simulink model "Sim3DoF"  (R2025b)
settings: Solver=VariableStepAuto  StartTime=0.0  StopTime=36  RelTol=1e-3
values from neighbouring files (symbols this model uses):
  hiddenLayerSizeCtrl = (2 * inputLayerSizeCtrl + 1) * 1    (= 13)    [Init2DoF.m]    (also in Init3DoF.m = 3)
  hiddenLayerSizeObsv = (2 * inputLayerSizeObsv + 1) * 1    (= 17)    [Init2DoF.m]    (also in Init3DoF.m = 3)
  n = 4    [Init2DoF.m]    (also in Init3DoF.m = 6)
  u_max = 12 * [1; 0.8]    [Init2DoF.m]    (also in Init3DoF.m = 25 * [1; 1; 1])
  u_min = - 12 * [1; 0.8]    [Init2DoF.m]    (also in Init3DoF.m = - 25 * [1; 1; 1])
  Vctrl0 = 0.1 * randn(hiddenLayerSizeCtrl, inputLayerSizeCtrl)    [Init2DoF.m]    (also in Init3DoF.m)
  Vobsv0 = 0.1 * randn(hiddenLayerSizeObsv, inputLayerSizeObsv)    [Init2DoF.m]    (also in Init3DoF.m)
  Wctrl0 = 0.1 * randn(outputLayerSizeCtrl, hiddenLayerSizeCtrl)    [Init2DoF.m]    (also in Init3DoF.m)
  Wobsv0 = 0.1 * randn(outputLayerSizeObsv, hiddenLayerSizeObsv)    [Init2DoF.m]    (also in Init3DoF.m)
  x0 = [0; 0.5; 0.1; 0]    [Init2DoF.m]    (also in Init3DoF.m = zeros(n, 1))
  x_hat0 = x0([1, 3, 2, 4])    [Init2DoF.m]    (also in Init3DoF.m = zeros(n, 1))
libraries: eeGeneralControl x2
settings Model: Creator=Asus  LastModifiedBy=Asus

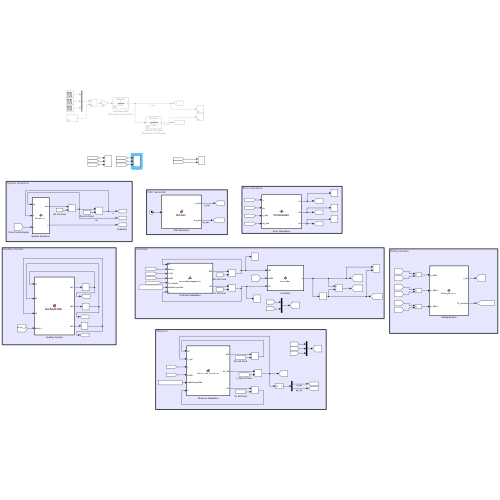
[thumbnail: Simulink's stored preview of the top-level diagram]
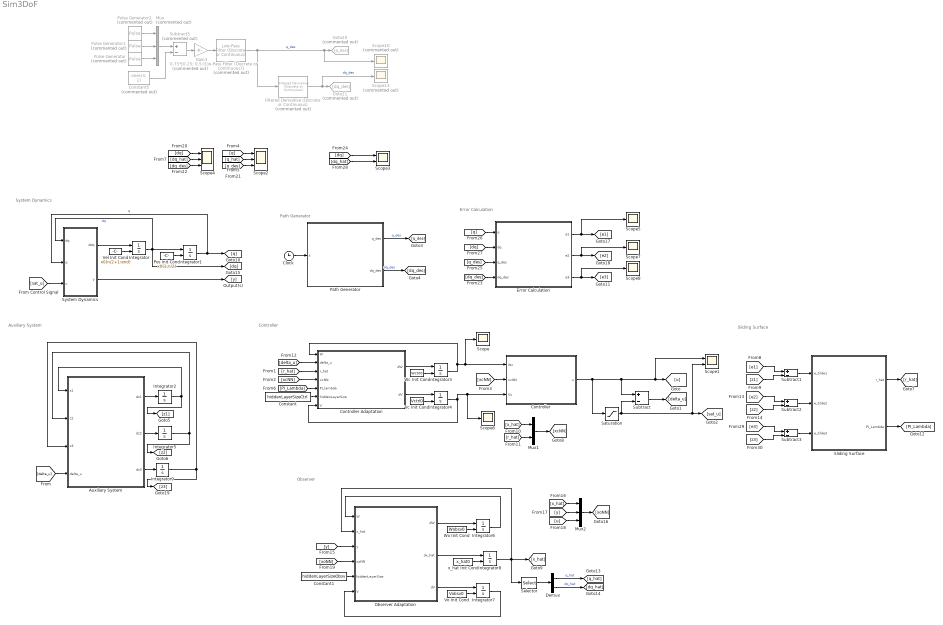
== system Sim3DoF ==
  note: System Dynamics
  note: Path Generator
  note: Auxiliary System
  note: Controller
  note: Sliding Surface
  note: Observer
  note: Error Calculation
  Auxiliary System : MATLAB Function  TreatAsAtomicUnit=on
  Clock : Clock
  Constant : Constant  Value=hiddenLayerSizeCtrl
  Constant1 : Constant  Value=hiddenLayerSizeObsv
  Constant5 : Constant  Commented=on  Value=ones(3, 1)
  Controller : MATLAB Function  TreatAsAtomicUnit=on
  Controller Adaptation : MATLAB Function  TreatAsAtomicUnit=on
  Demux : Demux  Outputs=2
  Error Calculation : MATLAB Function  TreatAsAtomicUnit=on
  Filtered Derivative (Discrete or Continuous) : eeGeneralControl/Filtered Derivative (Discrete or Continuous)  Commented=on  K=1  T=0.01  B=inf  A=-inf  minRatio=10  init_option=Inherited from block input  x0=0  Ts=-1
      settings: LibrarySourceBlock=|
      | ee_sl_lib/General Control/Filtered Derivative
      | (Discrete or Continuous)
  Gain3 : Gain  Commented=on  Gain=0.75*[0.25; 0.5; 1]
  Goto20 : Goto  Commented=on  GotoTag=q_des
  Goto21 : Goto  Commented=on  GotoTag=dq_des
  Integrator{,1,3..4,6..8} (7 alike) : Integrator  InitialConditionSource=external  InitialCondition=[0.5; 0.5]
  Integrator2 : Integrator  InitialCondition=zeros(2, 1)
  Integrator5 : Integrator  InitialCondition=zeros(2, 1)
  Integrator9 : Integrator  InitialCondition=zeros(2, 1)
  Low-Pass Filter (Discrete or Continuous)1 : eeGeneralControl/Low-Pass Filter (Discrete or Continuous)  Commented=on  K=1  T=0.5  B=inf  A=-inf  init_option=Inherited from block input  x0=0  Ts=-1
  Mux : Mux  Commented=on  Inputs=3
  Mux1 : Mux  Inputs=2
  Mux2 : Mux  Inputs=3
  Observer Adaptation : MATLAB Function  TreatAsAtomicUnit=on
  Path Generator : MATLAB Function  TreatAsAtomicUnit=on
  Pos Init Cond : Constant  Value=x0(1:n/2)
  Pulse Generator : DiscretePulseGenerator  Commented=on  PulseType=Time based  Amplitude=2  Period=14  PulseWidth=50
  Pulse Generator1 : DiscretePulseGenerator  Commented=on  PulseType=Time based  Amplitude=2  Period=16  PulseWidth=50
  Pulse Generator2 : DiscretePulseGenerator  Commented=on  PulseType=Time based  Amplitude=2  Period=18  PulseWidth=50
  Saturation : Saturate  UpperLimit=u_max  LowerLimit=u_min
  Scope{,5..8} (5 alike) : Scope
      Scope settings: ActiveDisplayYMinimum=-59.68968  ActiveDisplayYMaximum=12.0133
      Scope5 settings: ActiveDisplayYMinimum=-3.0151328940331377  ActiveDisplayYMaximum=1.4461258771147931
      Scope6 settings: ActiveDisplayYMinimum=-7.08799  ActiveDisplayYMaximum=6.5781  DataLoggingVariableName=ScopeData2
      Scope7 settings: ActiveDisplayYMinimum=-2.59713  ActiveDisplayYMaximum=1.51708  DataLoggingVariableName=ScopeData4
      Scope8 settings: ActiveDisplayYMinimum=-0.80491  ActiveDisplayYMaximum=2.91344
  Scope1 : Scope  NumInputPorts=2
      settings: ActiveDisplayYMinimum=-31.25  ActiveDisplayYMaximum=31.25
  Scope10 : Scope  Commented=on
      settings: ActiveDisplayYMinimum=-1  ActiveDisplayYMaximum=1  DataLoggingVariableName=ScopeData12
  Scope13 : Scope  Commented=on
      settings: ActiveDisplayYMinimum=-1  ActiveDisplayYMaximum=1  DataLoggingVariableName=ScopeData13
  Scope2 : Scope  NumInputPorts=3
      settings: ActiveDisplayYMinimum=-1.7944093115091528  ActiveDisplayYMaximum=1.8953759237714558
  Scope3 : Scope  NumInputPorts=2
      settings: ActiveDisplayYMinimum=-1.09542  ActiveDisplayYMaximum=0.61671  DataLoggingVariableName=ScopeData3
  Scope4 : Scope  NumInputPorts=3
      settings: ActiveDisplayYMinimum=-5.7037078996082133  ActiveDisplayYMaximum=15.052538924010589  DataLoggingVariableName=ScopeData2
  Selector : Selector  InputPortWidth=6  IndexOptions=Index vector (dialog)  Indices=[1, 3, 5, 2, 4, 6]  OutputSizes=1
  Sliding Surface : MATLAB Function  TreatAsAtomicUnit=on
  Subtract{,1..3} (4 alike) : Sum  Inputs=+-
  Subtract5 : Sum  Commented=on  Inputs=+-
  System Dynamics : MATLAB Function  TreatAsAtomicUnit=on
  Vc Init Cond : Constant  Value=Vctrl0
  Vel Init Cond : Constant  Value=x0(n/2+1:end)
  Vo Init Cond : Constant  Value=Vobsv0
  Wc Init Cond : Constant  Value=Wctrl0
  Wo Init Cond : Constant  Value=Wobsv0
  x_hat Init Cond : Constant  Value=x_hat0
  wires:
  [sat_u] -> System Dynamics/3(u)
  System Dynamics/1(ddq) -> Integrator/1
  System Dynamics/2(y) -> [y]
  Vel Init Cond/1 -> Integrator/2
  Pos Init Cond/1 -> Integrator1/2
  Clock/1 -> Path Generator/1(t)
  Auxiliary System/1(dz1) -> Integrator2/1
  Integrator2/1 -> [z1], Auxiliary System/1(z1)
  Controller/1(u) -> Saturation/1, Subtract/1, Scope1/1, [u]
  Wc Init Cond/1 -> Integrator3/2
  Controller Adaptation/1(dW) -> Integrator3/1
  Integrator3/1 -> Scope/1, Controller/1(Wc), Controller Adaptation/1(W)
  Controller Adaptation/2(dV) -> Integrator4/1
  Vc Init Cond/1 -> Integrator4/2
  Integrator4/1 -> Controller Adaptation/7(V), Scope6/1, Controller/3(Vc)
  [r_hat] -> Controller Adaptation/3(r_hat)
  [xcNN] -> Controller Adaptation/4(xcNN)
  [xcNN] -> Controller/2(xcNN)
  Auxiliary System/2(dz2) -> Integrator5/1
  Integrator5/1 -> [z2], Auxiliary System/2(z2)
  Mux1/1 -> [xcNN]
  [r_hat] -> Mux1/2
  Saturation/1 -> Scope1/2, [sat_u], Subtract/2
  [delta_u] -> Controller Adaptation/2(delta_u)
  Constant/1 -> Controller Adaptation/6(hiddenLayerSize)
  Sliding Surface/1(r_hat) -> [r_hat]
  [e1] -> Subtract1/1
  [z1] -> Subtract1/2
  Subtract1/1 -> Sliding Surface/1(e_tilde1)
  [z2] -> Subtract2/2
  [e2] -> Subtract2/1
  Subtract2/1 -> Sliding Surface/2(e_tilde2)
  Path Generator/2(dq_des) -> [dq_des]  "dq_des"
  Path Generator/1(q_des) -> [q_des]  "q_des"
  [q_hat] -> Scope2/2
  [PI_Lambda] -> Controller Adaptation/5(PI_lambda)
  Sliding Surface/2(PI_Lambda) -> [PI_Lambda]
  [dq_hat] -> Scope4/2
  Vo Init Cond/1 -> Integrator7/2
  Observer Adaptation/3(dV) -> Integrator7/1
  Wo Init Cond/1 -> Integrator6/2
  Integrator6/1 -> Observer Adaptation/1(W)
  Mux2/1 -> [xoNN]
  [y] -> Observer Adaptation/3(y)
  [xoNN] -> Observer Adaptation/4(xoNN)
  Integrator7/1 -> Observer Adaptation/6(V)
  Observer Adaptation/1(dW) -> Integrator6/1
  Constant1/1 -> Observer Adaptation/5(hiddenLayerSize)
  [u] -> Mux2/3
  [y] -> Mux2/2
  x_hat Init Cond/1 -> Integrator8/2
  Observer Adaptation/2(dx_hat) -> Integrator8/1
  [q_des] -> Scope2/3
  [dq_des] -> Scope4/3
  Integrator8/1 -> Selector/1, [x_hat], Observer Adaptation/2(x_hat)
  Error Calculation/2(e2) -> [e2], Scope7/1
  Error Calculation/1(e1) -> [e1], Scope5/1
  [q] -> Scope2/1
  [dq] -> Scope4/1
  [q] -> Error Calculation/1(q)
  [q_des] -> Error Calculation/3(q_des)
  [dq_des] -> Error Calculation/4(dq_des)
  [dq] -> Error Calculation/2(dq)
  [dq] -> Scope3/1
  [dq_hat] -> Scope3/2
  Demux/1 -> [q_hat]  "q_hat"
  Demux/2 -> [dq_hat]  "dq_hat"
  [x_hat] -> Mux2/1
  [x_hat] -> Mux1/1
  [delta_u] -> Auxiliary System/4(delta_u)
  Subtract/1 -> [delta_u]
  Integrator1/1 -> System Dynamics/2(q), [q]  "q"
  Integrator/1 -> [dq], Integrator1/1, System Dynamics/1(dq)  "dq"
  Error Calculation/3(e3) -> Scope8/1, [e3]
  Auxiliary System/3(dz3) -> Integrator9/1
  Integrator9/1 -> Auxiliary System/3(z3), [z3]
  [e3] -> Subtract3/1
  [z3] -> Subtract3/2
  Subtract3/1 -> Sliding Surface/3(e_tilde3)
  Selector/1 -> Demux/1
  Subtract5/1 -> Gain3/1
  Mux/1 -> Subtract5/1
  Gain3/1 -> Low-Pass Filter (Discrete or Continuous)1/1
  Low-Pass Filter (Discrete or Continuous)1/1 -> Filtered Derivative (Discrete or Continuous)/1, Scope10/1, Goto20/1  "q_des"
  Constant5/1 -> Subtract5/2
  Filtered Derivative (Discrete or Continuous)/1 -> Scope13/1, Goto21/1  "dq_des"
  Pulse Generator/1 -> Mux/3
  Pulse Generator2/1 -> Mux/1
  Pulse Generator1/1 -> Mux/2

== matlab function Sim3DoF/Observer Adaptation ==
  data: dW output; dx_hat output; dV output; W input; x_hat input; y input; xoNN input; hiddenLayerSize input; V input
function [dW, dx_hat, dV] = ObserverAdaptation(W, x_hat, y, xoNN, hiddenLayerSize, V)
    
    Sigma = @(z) (-1 + 2 ./ (1 + exp(-2 * z)));

    alpha = [2, 5; 2, 5; 2, 5];
    eps   = [0.1; 0.1; 0.1];

    A1ocl = [-alpha(1, 1)/eps(1), 1; -alpha(1, 2)/eps(1)^2, 0];
    A2ocl = [-alpha(2, 1)/eps(2), 1; -alpha(2, 2)/eps(2)^2, 0];
    A3ocl = [-alpha(3, 1)/eps(3), 1; -alpha(3, 2)/eps(3)^2, 0];
    B1    = [0; 1]; B2 = [0; 1]; B3 = [0; 1];
    C1    = [1; 0]; C2 = [1; 0]; C3 = [1; 0];

    Aocl  = blkdiag(A1ocl, A2ocl, A3ocl);
    B     = blkdiag(B1, B2, B3);
    C     = blkdiag(C1, C2, C3);

    A1o = [-alpha(1, 1)/eps(1), 1; 0, 0];
    A2o = [-alpha(2, 1)/eps(2), 1; 0, 0];
    A3o = [-alpha(3, 1)/eps(3), 1; 0, 0];
    Ao  = blkdiag(A1o, A2o, A3o);

    y_hat   = C' * x_hat;
    y_tilde = y - y_hat;

    rho1 = 2; rho2 = 2; rho3 = 2;
    Ho = [alpha(1, 2)/eps(1)^rho1 * y_tilde(1); alpha(2, 2)/eps(2)^rho2 * y_tilde(2); alpha(3, 2)/eps(3)^rho3 * y_tilde(3)];
    
    D1 = [alpha(1, 1)/eps(1); 0]; D2 = [alpha(2, 1)/eps(2); 0]; D3 = [alpha(3, 1)/eps(3); 0];
    D  = blkdiag(D1, D2, D3);

    psi_hat = W * Sigma(V * xoNN);
    dx_hat  = Ao * x_hat + B * (psi_hat + Ho) + D * y;

    eta   = [10, 10];
    gamma = [0.01, 0.01];

    PI_o = diag(Sigma(V * xoNN).^2);
    
    dW = - eta(1) * (y_tilde' * C' * Aocl^(-1) * B)' * Sigma(V * xoNN)' - gamma(1) * norm(y_tilde) * W;
    dV = - eta(2) * (y_tilde' * C' * Aocl^(-1) * B * W * (eye(hiddenLayerSize) - PI_o))' * xoNN' - gamma(2) * norm(y_tilde) * V;

end

== matlab function Sim3DoF/Error Calculation ==
  data: e1 output; e2 output; q input; dq input; q_des input; dq_des input; e3 output
function [e1, e2, e3] = ErrorCalculation(q, dq, q_des, dq_des)

    y_bar1 = [q(1); dq(1)];
    y_bar2 = [q(2); dq(2)];
    y_bar3 = [q(3); dq(3)];

    y_bar_des1 = [q_des(1); dq_des(1)];
    y_bar_des2 = [q_des(2); dq_des(2)];
    y_bar_des3 = [q_des(3); dq_des(3)];

    e1 = y_bar1 - y_bar_des1;
    e2 = y_bar2 - y_bar_des2;
    e3 = y_bar3 - y_bar_des3;
    
end

== matlab function Sim3DoF/Auxiliary System ==
  data: z1 input; z2 input; z3 input; dz1 output; delta_u input; dz2 output; dz3 output
function [dz1, dz2, dz3] = AuxiliarySystem(z1, z2, z3, delta_u)
    
    K1  = 15 * diag([-1, -2]); K2  = 15 * diag([-1, -2]); K3  = 15 * diag([-1, -2]);
    h1  = 15 * [-1; -2]; h2  = 15 * [-1; -2]; h3  = 15 * [-1; -2];

    dz1 = K1 * z1 + h1 * delta_u(1);
    dz2 = K2 * z2 + h2 * delta_u(2);
    dz3 = K3 * z3 + h3 * delta_u(3);
    
end

== matlab function Sim3DoF/System Dynamics ==
  data: dq input; q input; ddq output; y output; u input
function [ddq, y] = Dynamics(dq, q, u)

    M = [                                                                                               (cos(q(1))*cos(q(2)) + (cos(q(1))*cos(q(2))*cos(q(3)))/2 - (cos(q(1))*sin(q(2))*sin(q(3)))/2)^2 + (cos(q(1))^2*cos(q(2))^2)/4 + (cos(q(2))*sin(q(1)) - (sin(q(1))*sin(q(2))*sin(q(3)))/2 + (cos(q(2))*cos(q(3))*sin(q(1)))/2)^2 + (cos(q(2))^2*sin(q(1))^2)/4 + 1/4,                                                                                               (cos(q(1))*sin(q(2)) + (cos(q(1))*cos(q(2))*sin(q(3)))/2 + (cos(q(1))*cos(q(3))*sin(q(2)))/2)*(cos(q(2))*sin(q(1)) - (sin(q(1))*sin(q(2))*sin(q(3)))/2 + (cos(q(2))*cos(q(3))*sin(q(1)))/2) - (cos(q(1))*cos(q(2)) + (cos(q(1))*cos(q(2))*cos(q(3)))/2 - (cos(q(1))*sin(q(2))*sin(q(3)))/2)*(sin(q(1))*sin(q(2)) + (cos(q(2))*sin(q(1))*sin(q(3)))/2 + (cos(q(3))*sin(q(1))*sin(q(2)))/2),                                                                                                                                   ((cos(q(1))*cos(q(2))*sin(q(3)))/2 + (cos(q(1))*cos(q(3))*sin(q(2)))/2)*(cos(q(2))*sin(q(1)) - (sin(q(1))*sin(q(2))*sin(q(3)))/2 + (cos(q(2))*cos(q(3))*sin(q(1)))/2) - ((cos(q(2))*sin(q(1))*sin(q(3)))/2 + (cos(q(3))*sin(q(1))*sin(q(2)))/2)*(cos(q(1))*cos(q(2)) + (cos(q(1))*cos(q(2))*cos(q(3)))/2 - (cos(q(1))*sin(q(2))*sin(q(3)))/2)
    (cos(q(1))*sin(q(2)) + (cos(q(1))*cos(q(2))*sin(q(3)))/2 + (cos(q(1))*cos(q(3))*sin(q(2)))/2)*(cos(q(2))*sin(q(1)) - (sin(q(1))*sin(q(2))*sin(q(3)))/2 + (cos(q(2))*cos(q(3))*sin(q(1)))/2) - (cos(q(1))*cos(q(2)) + (cos(q(1))*cos(q(2))*cos(q(3)))/2 - (cos(q(1))*sin(q(2))*sin(q(3)))/2)*(sin(q(1))*sin(q(2)) + (cos(q(2))*sin(q(1))*sin(q(3)))/2 + (cos(q(3))*sin(q(1))*sin(q(2)))/2),                                                                                               cos(q(1))^2/6 + cos(q(2))^2/4 + sin(q(1))^2/6 + (cos(q(1))*sin(q(2)) + (cos(q(1))*cos(q(2))*sin(q(3)))/2 + (cos(q(1))*cos(q(3))*sin(q(2)))/2)^2 + (cos(q(2)) + (cos(q(2))*cos(q(3)))/2 - (sin(q(2))*sin(q(3)))/2)^2 + (cos(q(1))^2*sin(q(2))^2)/4 + (sin(q(1))*sin(q(2)) + (cos(q(2))*sin(q(1))*sin(q(3)))/2 + (cos(q(3))*sin(q(1))*sin(q(2)))/2)^2 + (sin(q(1))^2*sin(q(2))^2)/4, cos(q(1))^2/12 + ((cos(q(2))*sin(q(1))*sin(q(3)))/2 + (cos(q(3))*sin(q(1))*sin(q(2)))/2)*(sin(q(1))*sin(q(2)) + (cos(q(2))*sin(q(1))*sin(q(3)))/2 + (cos(q(3))*sin(q(1))*sin(q(2)))/2) + sin(q(1))^2/12 + ((cos(q(2))*cos(q(3)))/2 - (sin(q(2))*sin(q(3)))/2)*(cos(q(2)) + (cos(q(2))*cos(q(3)))/2 - (sin(q(2))*sin(q(3)))/2) + ((cos(q(1))*cos(q(2))*sin(q(3)))/2 + (cos(q(1))*cos(q(3))*sin(q(2)))/2)*(cos(q(1))*sin(q(2)) + (cos(q(1))*cos(q(2))*sin(q(3)))/2 + (cos(q(1))*cos(q(3))*sin(q(2)))/2)
    ((cos(q(1))*cos(q(2))*sin(q(3)))/2 + (cos(q(1))*cos(q(3))*sin(q(2)))/2)*(cos(q(2))*sin(q(1)) - (sin(q(1))*sin(q(2))*sin(q(3)))/2 + (cos(q(2))*cos(q(3))*sin(q(1)))/2) - ((cos(q(2))*sin(q(1))*sin(q(3)))/2 + (cos(q(3))*sin(q(1))*sin(q(2)))/2)*(cos(q(1))*cos(q(2)) + (cos(q(1))*cos(q(2))*cos(q(3)))/2 - (cos(q(1))*sin(q(2))*sin(q(3)))/2), cos(q(1))^2/12 + ((cos(q(2))*sin(q(1))*sin(q(3)))/2 + (cos(q(3))*sin(q(1))*sin(q(2)))/2)*(sin(q(1))*sin(q(2)) + (cos(q(2))*sin(q(1))*sin(q(3)))/2 + (cos(q(3))*sin(q(1))*sin(q(2)))/2) + sin(q(1))^2/12 + ((cos(q(2))*cos(q(3)))/2 - (sin(q(2))*sin(q(3)))/2)*(cos(q(2)) + (cos(q(2))*cos(q(3)))/2 - (sin(q(2))*sin(q(3)))/2) + ((cos(q(1))*cos(q(2))*sin(q(3)))/2 + (cos(q(1))*cos(q(3))*sin(q(2)))/2)*(cos(q(1))*sin(q(2)) + (cos(q(1))*cos(q(2))*sin(q(3)))/2 + (cos(q(1))*cos(q(3))*sin(q(2)))/2),                                                                                                                                                                                                             cos(q(1))^2/12 + sin(q(1))^2/12 + ((cos(q(1))*cos(q(2))*sin(q(3)))/2 + (cos(q(1))*cos(q(3))*sin(q(2)))/2)^2 + ((cos(q(2))*sin(q(1))*sin(q(3)))/2 + (cos(q(3))*sin(q(1))*sin(q(2)))/2)^2 + ((cos(q(2))*cos(q(3)))/2 - (sin(q(2))*sin(q(3)))/2)^2];


    C = [ - dq(2)*((cos(q(2))*sin(q(1)) - (sin(q(1))*sin(q(2))*sin(q(3)))/2 + (cos(q(2))*cos(q(3))*sin(q(1)))/2)*(sin(q(1))*sin(q(2)) + (cos(q(2))*sin(q(1))*sin(q(3)))/2 + (cos(q(3))*sin(q(1))*sin(q(2)))/2) + (cos(q(1))*cos(q(2)) + (cos(q(1))*cos(q(2))*cos(q(3)))/2 - (cos(q(1))*sin(q(2))*sin(q(3)))/2)*(cos(q(1))*sin(q(2)) + (cos(q(1))*cos(q(2))*sin(q(3)))/2 + (cos(q(1))*cos(q(3))*sin(q(2)))/2) + (cos(q(1))^2*cos(q(2))*sin(q(2)))/4 + (cos(q(2))*sin(q(1))^2*sin(q(2)))/4) - dq(3)*(((cos(q(2))*sin(q(1))*sin(q(3)))/2 + (cos(q(3))*sin(q(1))*sin(q(2)))/2)*(cos(q(2))*sin(q(1)) - (sin(q(1))*sin(q(2))*sin(q(3)))/2 + (cos(q(2))*cos(q(3))*sin(q(1)))/2) + ((cos(q(1))*cos(q(2))*sin(q(3)))/2 + (cos(q(1))*cos(q(3))*sin(q(2)))/2)*(cos(q(1))*cos(q(2)) + (cos(q(1))*cos(q(2))*cos(q(3)))/2 - (cos(q(1))*sin(q(2))*sin(q(3)))/2)),                                                                                                                                                                                                                                                                                                                                                     dq(3)*(((cos(q(1))*cos(q(2))*cos(q(3)))/2 - (cos(q(1))*sin(q(2))*sin(q(3)))/2)*(cos(q(2))*sin(q(1)) - (sin(q(1))*sin(q(2))*sin(q(3)))/2 + (cos(q(2))*cos(q(3))*sin(q(1)))/2) + ((sin(q(1))*sin(q(2))*sin(q(3)))/2 - (cos(q(2))*cos(q(3))*sin(q(1)))/2)*(cos(q(1))*cos(q(2)) + (cos(q(1))*cos(q(2))*cos(q(3)))/2 - (cos(q(1))*sin(q(2))*sin(q(3)))/2)) - dq(1)*((cos(q(2))*sin(q(1)) - (sin(q(1))*sin(q(2))*sin(q(3)))/2 + (cos(q(2))*cos(q(3))*sin(q(1)))/2)*(sin(q(1))*sin(q(2)) + (cos(q(2))*sin(q(1))*sin(q(3)))/2 + (cos(q(3))*sin(q(1))*sin(q(2)))/2) + (cos(q(1))*cos(q(2)) + (cos(q(1))*cos(q(2))*cos(q(3)))/2 - (cos(q(1))*sin(q(2))*sin(q(3)))/2)*(cos(q(1))*sin(q(2)) + (cos(q(1))*cos(q(2))*sin(q(3)))/2 + (cos(q(1))*cos(q(3))*sin(q(2)))/2) + (cos(q(1))^2*cos(q(2))*sin(q(2)))/4 + (cos(q(2))*sin(q(1))^2*sin(q(2)))/4),                                                                                                                                                                                                           dq(2)*(((cos(q(1))*cos(q(2))*cos(q(3)))/2 - (cos(q(1))*sin(q(2))*sin(q(3)))/2)*(cos(q(2))*sin(q(1)) - (sin(q(1))*sin(q(2))*sin(q(3)))/2 + (cos(q(2))*cos(q(3))*sin(q(1)))/2) + ((sin(q(1))*sin(q(2))*sin(q(3)))/2 - (cos(q(2))*cos(q(3))*sin(q(1)))/2)*(cos(q(1))*cos(q(2)) + (cos(q(1))*cos(q(2))*cos(q(3)))/2 - (cos(q(1))*sin(q(2))*sin(q(3)))/2)) - dq(1)*(((cos(q(2))*sin(q(1))*sin(q(3)))/2 + (cos(q(3))*sin(q(1))*sin(q(2)))/2)*(cos(q(2))*sin(q(1)) - (sin(q(1))*sin(q(2))*sin(q(3)))/2 + (cos(q(2))*cos(q(3))*sin(q(1)))/2) + ((cos(q(1))*cos(q(2))*sin(q(3)))/2 + (cos(q(1))*cos(q(3))*sin(q(2)))/2)*(cos(q(1))*cos(q(2)) + (cos(q(1))*cos(q(2))*cos(q(3)))/2 - (cos(q(1))*sin(q(2))*sin(q(3)))/2)) + dq(3)*(((cos(q(1))*cos(q(2))*cos(q(3)))/2 - (cos(q(1))*sin(q(2))*sin(q(3)))/2)*(cos(q(2))*sin(q(1)) - (sin(q(1))*sin(q(2))*sin(q(3)))/2 + (cos(q(2))*cos(q(3))*sin(q(1)))/2) + ((sin(q(1))*sin(q(2))*sin(q(3)))/2 - (cos(q(2))*cos(q(3))*sin(q(1)))/2)*(cos(q(1))*cos(q(2)) + (cos(q(1))*cos(q(2))*cos(q(3)))/2 - (cos(q(1))*sin(q(2))*sin(q(3)))/2))
        dq(1)*((cos(q(2))*sin(q(1)) - (sin(q(1))*sin(q(2))*sin(q(3)))/2 + (cos(q(2))*cos(q(3))*sin(q(1)))/2)*(sin(q(1))*sin(q(2)) + (cos(q(2))*sin(q(1))*sin(q(3)))/2 + (cos(q(3))*sin(q(1))*sin(q(2)))/2) + (cos(q(1))*cos(q(2)) + (cos(q(1))*cos(q(2))*cos(q(3)))/2 - (cos(q(1))*sin(q(2))*sin(q(3)))/2)*(cos(q(1))*sin(q(2)) + (cos(q(1))*cos(q(2))*sin(q(3)))/2 + (cos(q(1))*cos(q(3))*sin(q(2)))/2) + (cos(q(1))^2*cos(q(2))*sin(q(2)))/4 + (cos(q(2))*sin(q(1))^2*sin(q(2)))/4) - dq(3)*(((cos(q(2))*sin(q(1))*sin(q(3)))/2 + (cos(q(3))*sin(q(1))*sin(q(2)))/2)*(cos(q(1))*sin(q(2)) + (cos(q(1))*cos(q(2))*sin(q(3)))/2 + (cos(q(1))*cos(q(3))*sin(q(2)))/2) - ((cos(q(1))*cos(q(2))*sin(q(3)))/2 + (cos(q(1))*cos(q(3))*sin(q(2)))/2)*(sin(q(1))*sin(q(2)) + (cos(q(2))*sin(q(1))*sin(q(3)))/2 + (cos(q(3))*sin(q(1))*sin(q(2)))/2)),                                                                                                             dq(2)*((cos(q(2))*sin(q(1)) - (sin(q(1))*sin(q(2))*sin(q(3)))/2 + (cos(q(2))*cos(q(3))*sin(q(1)))/2)*(sin(q(1))*sin(q(2)) + (cos(q(2))*sin(q(1))*sin(q(3)))/2 + (cos(q(3))*sin(q(1))*sin(q(2)))/2) - (cos(q(2)) + (cos(q(2))*cos(q(3)))/2 - (sin(q(2))*sin(q(3)))/2)*(sin(q(2)) + (cos(q(2))*sin(q(3)))/2 + (cos(q(3))*sin(q(2)))/2) - (cos(q(2))*sin(q(2)))/4 + (cos(q(1))*cos(q(2)) + (cos(q(1))*cos(q(2))*cos(q(3)))/2 - (cos(q(1))*sin(q(2))*sin(q(3)))/2)*(cos(q(1))*sin(q(2)) + (cos(q(1))*cos(q(2))*sin(q(3)))/2 + (cos(q(1))*cos(q(3))*sin(q(2)))/2) + (cos(q(1))^2*cos(q(2))*sin(q(2)))/4 + (cos(q(2))*sin(q(1))^2*sin(q(2)))/4) - dq(3)*(((sin(q(1))*sin(q(2))*sin(q(3)))/2 - (cos(q(2))*cos(q(3))*sin(q(1)))/2)*(sin(q(1))*sin(q(2)) + (cos(q(2))*sin(q(1))*sin(q(3)))/2 + (cos(q(3))*sin(q(1))*sin(q(2)))/2) + ((cos(q(2))*sin(q(3)))/2 + (cos(q(3))*sin(q(2)))/2)*(cos(q(2)) + (cos(q(2))*cos(q(3)))/2 - (sin(q(2))*sin(q(3)))/2) - ((cos(q(1))*cos(q(2))*cos(q(3)))/2 - (cos(q(1))*sin(q(2))*sin(q(3)))/2)*(cos(q(1))*sin(q(2)) + (cos(q(1))*cos(q(2))*sin(q(3)))/2 + (cos(q(1))*cos(q(3))*sin(q(2)))/2)), - dq(1)*(((cos(q(2))*sin(q(1))*sin(q(3)))/2 + (cos(q(3))*sin(q(1))*sin(q(2)))/2)*(cos(q(1))*sin(q(2)) + (cos(q(1))*cos(q(2))*sin(q(3)))/2 + (cos(q(1))*cos(q(3))*sin(q(2)))/2) - ((cos(q(1))*cos(q(2))*sin(q(3)))/2 + (cos(q(1))*cos(q(3))*sin(q(2)))/2)*(sin(q(1))*sin(q(2)) + (cos(q(2))*sin(q(1))*sin(q(3)))/2 + (cos(q(3))*sin(q(1))*sin(q(2)))/2)) - dq(2)*(((sin(q(1))*sin(q(2))*sin(q(3)))/2 - (cos(q(2))*cos(q(3))*sin(q(1)))/2)*(sin(q(1))*sin(q(2)) + (cos(q(2))*sin(q(1))*sin(q(3)))/2 + (cos(q(3))*sin(q(1))*sin(q(2)))/2) + ((cos(q(2))*sin(q(3)))/2 + (cos(q(3))*sin(q(2)))/2)*(cos(q(2)) + (cos(q(2))*cos(q(3)))/2 - (sin(q(2))*sin(q(3)))/2) - ((cos(q(1))*cos(q(2))*cos(q(3)))/2 - (cos(q(1))*sin(q(2))*sin(q(3)))/2)*(cos(q(1))*sin(q(2)) + (cos(q(1))*cos(q(2))*sin(q(3)))/2 + (cos(q(1))*cos(q(3))*sin(q(2)))/2)) - dq(3)*(((sin(q(1))*sin(q(2))*sin(q(3)))/2 - (cos(q(2))*cos(q(3))*sin(q(1)))/2)*(sin(q(1))*sin(q(2)) + (cos(q(2))*sin(q(1))*sin(q(3)))/2 + (cos(q(3))*sin(q(1))*sin(q(2)))/2) + ((cos(q(2))*sin(q(3)))/2 + (cos(q(3))*sin(q(2)))/2)*(cos(q(2)) + (cos(q(2))*cos(q(3)))/2 - (sin(q(2))*sin(q(3)))/2) - ((cos(q(1))*cos(q(2))*cos(q(3)))/2 - (cos(q(1))*sin(q(2))*sin(q(3)))/2)*(cos(q(1))*sin(q(2)) + (cos(q(1))*cos(q(2))*sin(q(3)))/2 + (cos(q(1))*cos(q(3))*sin(q(2)))/2))
        dq(1)*(((cos(q(2))*sin(q(1))*sin(q(3)))/2 + (cos(q(3))*sin(q(1))*sin(q(2)))/2)*(cos(q(2))*sin(q(1)) - (sin(q(1))*sin(q(2))*sin(q(3)))/2 + (cos(q(2))*cos(q(3))*sin(q(1)))/2) + ((cos(q(1))*cos(q(2))*sin(q(3)))/2 + (cos(q(1))*cos(q(3))*sin(q(2)))/2)*(cos(q(1))*cos(q(2)) + (cos(q(1))*cos(q(2))*cos(q(3)))/2 - (cos(q(1))*sin(q(2))*sin(q(3)))/2)) + dq(2)*(((cos(q(2))*sin(q(1))*sin(q(3)))/2 + (cos(q(3))*sin(q(1))*sin(q(2)))/2)*(cos(q(1))*sin(q(2)) + (cos(q(1))*cos(q(2))*sin(q(3)))/2 + (cos(q(1))*cos(q(3))*sin(q(2)))/2) - ((cos(q(1))*cos(q(2))*sin(q(3)))/2 + (cos(q(1))*cos(q(3))*sin(q(2)))/2)*(sin(q(1))*sin(q(2)) + (cos(q(2))*sin(q(1))*sin(q(3)))/2 + (cos(q(3))*sin(q(1))*sin(q(2)))/2)), dq(1)*(((cos(q(2))*sin(q(1))*sin(q(3)))/2 + (cos(q(3))*sin(q(1))*sin(q(2)))/2)*(cos(q(1))*sin(q(2)) + (cos(q(1))*cos(q(2))*sin(q(3)))/2 + (cos(q(1))*cos(q(3))*sin(q(2)))/2) - ((cos(q(1))*cos(q(2))*sin(q(3)))/2 + (cos(q(1))*cos(q(3))*sin(q(2)))/2)*(sin(q(1))*sin(q(2)) + (cos(q(2))*sin(q(1))*sin(q(3)))/2 + (cos(q(3))*sin(q(1))*sin(q(2)))/2)) - dq(3)*(((sin(q(1))*sin(q(2))*sin(q(3)))/2 - (cos(q(2))*cos(q(3))*sin(q(1)))/2)*((cos(q(2))*sin(q(1))*sin(q(3)))/2 + (cos(q(3))*sin(q(1))*sin(q(2)))/2) + ((cos(q(2))*cos(q(3)))/2 - (sin(q(2))*sin(q(3)))/2)*((cos(q(2))*sin(q(3)))/2 + (cos(q(3))*sin(q(2)))/2) - ((cos(q(1))*cos(q(2))*cos(q(3)))/2 - (cos(q(1))*sin(q(2))*sin(q(3)))/2)*((cos(q(1))*cos(q(2))*sin(q(3)))/2 + (cos(q(1))*cos(q(3))*sin(q(2)))/2)) + dq(2)*(((cos(q(2))*sin(q(1))*sin(q(3)))/2 + (cos(q(3))*sin(q(1))*sin(q(2)))/2)*(cos(q(2))*sin(q(1)) - (sin(q(1))*sin(q(2))*sin(q(3)))/2 + (cos(q(2))*cos(q(3))*sin(q(1)))/2) - ((cos(q(2))*cos(q(3)))/2 - (sin(q(2))*sin(q(3)))/2)*(sin(q(2)) + (cos(q(2))*sin(q(3)))/2 + (cos(q(3))*sin(q(2)))/2) + ((cos(q(1))*cos(q(2))*sin(q(3)))/2 + (cos(q(1))*cos(q(3))*sin(q(2)))/2)*(cos(q(1))*cos(q(2)) + (cos(q(1))*cos(q(2))*cos(q(3)))/2 - (cos(q(1))*sin(q(2))*sin(q(3)))/2)),                                                                                                                                                                                                                                                                                                                                                                                           - dq(2)*(((sin(q(1))*sin(q(2))*sin(q(3)))/2 - (cos(q(2))*cos(q(3))*sin(q(1)))/2)*((cos(q(2))*sin(q(1))*sin(q(3)))/2 + (cos(q(3))*sin(q(1))*sin(q(2)))/2) + ((cos(q(2))*cos(q(3)))/2 - (sin(q(2))*sin(q(3)))/2)*((cos(q(2))*sin(q(3)))/2 + (cos(q(3))*sin(q(2)))/2) - ((cos(q(1))*cos(q(2))*cos(q(3)))/2 - (cos(q(1))*sin(q(2))*sin(q(3)))/2)*((cos(q(1))*cos(q(2))*sin(q(3)))/2 + (cos(q(1))*cos(q(3))*sin(q(2)))/2)) - dq(3)*(((sin(q(1))*sin(q(2))*sin(q(3)))/2 - (cos(q(2))*cos(q(3))*sin(q(1)))/2)*((cos(q(2))*sin(q(1))*sin(q(3)))/2 + (cos(q(3))*sin(q(1))*sin(q(2)))/2) + ((cos(q(2))*cos(q(3)))/2 - (sin(q(2))*sin(q(3)))/2)*((cos(q(2))*sin(q(3)))/2 + (cos(q(3))*sin(q(2)))/2) - ((cos(q(1))*cos(q(2))*cos(q(3)))/2 - (cos(q(1))*sin(q(2))*sin(q(3)))/2)*((cos(q(1))*cos(q(2))*sin(q(3)))/2 + (cos(q(1))*cos(q(3))*sin(q(2)))/2))];
    
    G =  [           0
        (981*cos(q(2) + q(3)))/200 + (2943*cos(q(2)))/200
        (981*cos(q(2) + q(3)))/200];
    
    % robot dynamics
    ddq = M \ (u - C * dq - G);
    y   = q;
    
end

== matlab function Sim3DoF/Path Generator ==
  data: t input; q_des output; dq_des output
function [q_des, dq_des] = PathGen(t)
    
    w = 0.2;
    A = 0.5;

    q_des   = A *       [ sin(w*t);  cos(w*t); sin(w*t + pi/3)];
    dq_des  = A * w *   [ cos(w*t); -sin(w*t); cos(w*t + pi/3)];
    % ddq_des = A * w^2 * [-sin(w*t); -cos(w*t); -sin(w*t) - cos(w*t)];

    
end

== matlab function Sim3DoF/Controller ==
  data: u output; Wc input; xcNN input; Vc input
function u = Controller(Wc, xcNN, Vc)

    Sigma = @(z) (-1 + 2 ./ (1 + exp(-2 * z)));

    u = - Wc * Sigma(Vc * xcNN);
    
end

== matlab function Sim3DoF/Controller Adaptation ==
  data: dW output; dV output; W input; delta_u input; r_hat input; xcNN input; PI_lambda input; hiddenLayerSize input; V input
function [dW, dV] = ControllerAdaptation(W, delta_u, r_hat, xcNN, PI_lambda, hiddenLayerSize, V)
    
    Sigma = @(z) (-1 + 2 ./ (1 + exp(-2 * z)));

    Ac1 = [0, 1; -0.01, -0.2]; B1 = [0; 1];
    Ac2 = [0, 1; -0.01, -0.2]; B2 = [0; 1];
    Ac3 = [0, 1; -0.01, -0.2]; B3 = [0; 1];
    
    Ac = blkdiag(Ac1, Ac2, Ac3);
    B  = blkdiag(B1, B2, B3);

    K1  = 15 * diag([-1, -2]); K2  = 15 * diag([-1, -2]); K3  = 15 * diag([-1, -2]);
    K  = blkdiag(K1, K2, K3);

    h1  = 15 * [-1; -2]; h2  = 15 * [-1; -2]; h3  = 15 * [-1; -2];
    h  = blkdiag(h1, h2, h3); % bug potential

    eta   = [0.1, 0.1];
    gamma = [0.001, 0.001];

    PI_c = diag(Sigma(V * xcNN).^2);
    
    dW = eta(1) * (r_hat' * PI_lambda * (-Ac^(-1) * B + K^(-1) * h * diag(delta_u)))' * Sigma(V * xcNN)' - gamma(1) * norm(r_hat) * W;
    dV = eta(2) * (r_hat' * PI_lambda * (-Ac^(-1) * B + K^(-1) * h * diag(delta_u)) * W * (eye(hiddenLayerSize) - PI_c))' * xcNN' - gamma(2) * norm(r_hat) * V;

end

== matlab function Sim3DoF/Sliding Surface ==
  data: e_tilde1 input; r_hat output; e_tilde2 input; PI_Lambda output; e_tilde3 input
function [r_hat, PI_Lambda] = SlidingSurface(e_tilde1, e_tilde2, e_tilde3)

    Lambda1 = 5; Lambda2 = 5; Lambda3 = 5;

    r_hat1  = [Lambda1, 1] * e_tilde1;
    r_hat2  = [Lambda2, 1] * e_tilde2;
    r_hat3  = [Lambda3, 1] * e_tilde3;

    r_hat   = [r_hat1; r_hat2; r_hat3];

    PI_Lambda = blkdiag([Lambda1, 1], [Lambda2, 1], [Lambda3, 1]);
    
end
